simulink model "OFDM"  (R2022b)
settings: Solver=FixedStepDiscrete  StartTime=0.0  StopTime=inf  RelTol=1e-3
PreLoadFcn:
  | init
InitFcn:
  | init
values from neighbouring files (symbols this model uses):
  M = 3    [init.m]
  N = 2048    [init.m]
  nbPilots = 32    [init.m]
  nbZeros = N/8    (= 256)    [init.m]    (also in tests.m = N/8)
  nCycle = delayMax * N / Ts    (= 2)    [init.m]    (also in setMyParams.m = delaymax * n / Ts)
  nTotal = N + nCycle    (= 2050)    [init.m]    (also in setMyParams.m = n + nCycle)
  nUtile = N - ( nbZeros + nbPilots )    (= 1760)    [init.m]    (also in setMyParams.m = n - ( nbzeros + nbpilots ))
  Ts = N/B    (= 0.0001024)    [init.m]    (also in setMyParams.m = n/b)
undefined symbols (not defined in the file or in its folder): doppler, PSK
libraries: commchan3 x2, simulink x2, dspxfrm3 x2, commdigbbndam3 x2, commrandsrc3 x1, commsink2 x1
settings Model: SimulationMode=accelerator  Creator=pchabance  LastModifiedBy=AIIH
settings SolverCC: AlgebraicLoopSolver=TrustRegion  AutoInsertRateTranBlk=on
settings DataIOCC: LimitDataPoints=on  SaveOutput=off  SignalLogging=off  SaveTime=off  ReturnWorkspaceOutputs=off
settings OptimizationCC: EfficientMapNaN2IntZero=off  LifeSpan=inf
settings DebuggingCC: AlgebraicLoopMsg=error  SingleTaskRateTransMsg=error  UnconnectedInputMsg=warning  UnconnectedOutputMsg=warning  UnconnectedLineMsg=warning  AllowSymbolicDim=off  SFUnexpectedBacktrackingDiag=warning  SFNoUnconditionalDefaultTransitionDiag=warning  SFExecutionAtInitializationDiag=none  SFMachineParentedDataDiag=warning  ArithmeticOperatorsInVariantConditions=warning
settings HardwareCC: TargetBitPerPointer=64  TargetBitPerSizeT=64  TargetBitPerPtrDiffT=64  TargetLongLongMode=on  TargetIntDivRoundTo=Zero  TargetEndianess=LittleEndian  TargetWordSize=64  TargetHWDeviceType=MATLAB Host  ProdEqTarget=off
settings ModelReferenceCC: EnableRefExpFcnMdlSchedulingChecks=on
settings SFSimCC: SimUseLocalCustomCode=off  CustomCodeUndefinedFunction=UseInterfaceOnly
settings RTWCC: RTWUseLocalCustomCode=off
settings CodeAppCC: MaxIdLength=128  StateflowObjectComments=on
settings GRTTargetCC: TargetLangStandard=C89/C90 (ANSI)  CombineOutputUpdateFcns=off  GRTInterface=on

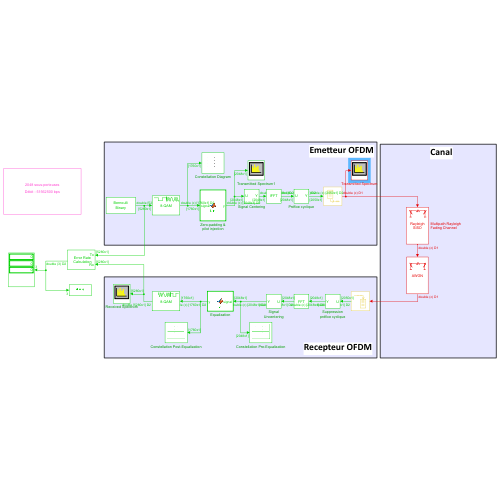
[thumbnail: Simulink's stored preview of the top-level diagram]
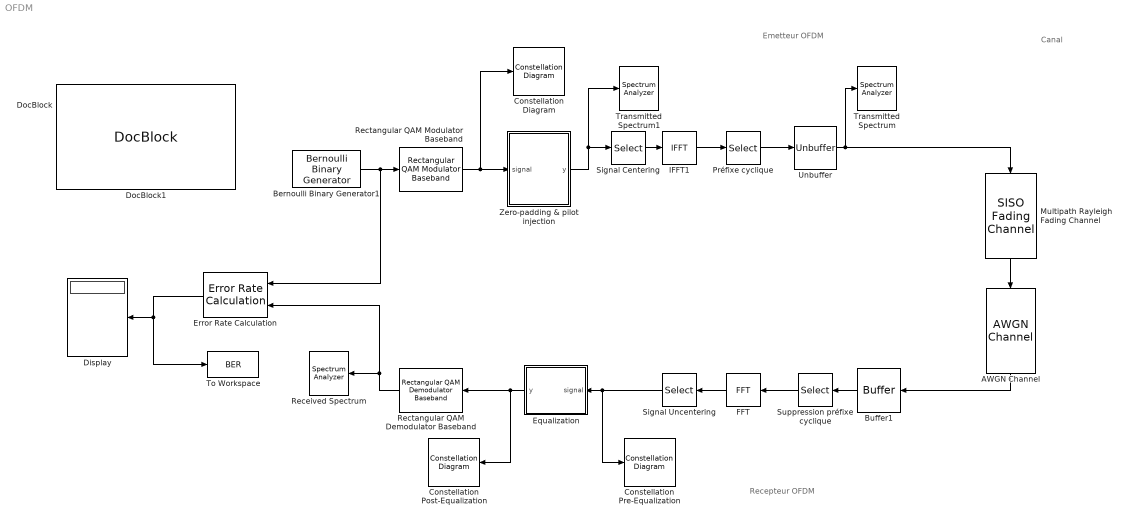
== system OFDM ==
  note: Emetteur OFDM
  note: Recepteur OFDM
  note: Canal
  AWGN Channel : commchan3/AWGN Channel  InputProcessing=Columns as channels (frame based)  seed=67  noiseMode="Signal to noise ratio  (SNR)"  EbNodB=10  EsNodB=30  SNRdB=SNR_  bitsPerSym=2  Ps=W  Tsym=256*5e-8  variance=1
  Bernoulli Binary Generator1 : commrandsrc3/Bernoulli Binary Generator  ProbabilityOfZero=0.5  SeedSource=Auto  Seed=0  SampleTime=Ts/(nUtile*M)  SamplesPerFrame=nUtile*M  OutputDataType=double  SimulateUsing=Code generation
  Buffer1 : Buffer  N=nTotal  OutputFrames=off
  Constellation Diagram : ConstellationDiagram  WindowPosition=[433.000000,362.000000,410.000000,300.000000,]  Visible=on  ScopeFrameLocation=window  DefaultConfigurationName=comm.scopes.ConstellationDiagramBlockCfg
  Constellation Post-Equalization : ConstellationDiagram  WindowPosition=[388.000000,174.000000,422.000000,306.000000,]  Visible=on  ScopeFrameLocation=window  SymbolsToDisplaySource=Property  SymbolsToDisplay=8000  ReferenceConstellation=8-PSK  XLimits=[-1.596 1.5905]  YLimits=[-1.9943 1.9888]  DefaultConfigurationName=comm.scopes.ConstellationDiagramBlockCfg
  Constellation Pre-Equalization : ConstellationDiagram  WindowPosition=[1.000000,26.000000,1280.000000,844.000000,]  Visible=on  ScopeFrameLocation=window  ReferenceConstellation=8-PSK  XLimits=[-2.0473 1.1549]  YLimits=[-2.4475 1.5551]  DefaultConfigurationName=comm.scopes.ConstellationDiagramBlockCfg
  Display : Display
  DocBlock : simulink/Model-Wide Utilities/DocBlock  DocumentType=Text
      content=|
      | Type your documentation here
  DocBlock1 : simulink/Model-Wide Utilities/DocBlock  DocumentType=Text  mask(DocBlock){}
      content=|
      | Type your documentation here
      mask Display:
      | % This is a new mask on top of the base mask.
      | % Use "View base mask" link below to see the base mask.
      | 
      | N = evalin('base','N');
      | fprintf([num2str(N),' sous-porteuses\n\n\n']);
      | 
      | rate = evalin('base','debit');
      | fprintf(['Débit : ',num2str(rate),' bps']);
  Equalization : MATLAB Function  TreatAsAtomicUnit=on
  Error Rate Calculation : commsink2/Error Rate Calculation  N=nUtile*M  st_delay=0  cp_mode=Entire frame  subframe=[]  PMode=Port  WsName=ErrorVec  RsMode2=off  stop=off  numErr=100  maxBits=1e6
  FFT : dspxfrm3/FFT  FFTImplementation=Auto  CompMethod=Table lookup  TableOpt=NEW  TableOptActive=Speed  BitRevOrder=off  Normalize=off  InheritFFTLength=on  FFTLength=64  WrapInput=on  roundingMode=Floor  overflowMode=off  firstCoeffDataTypeStr=Inherit: Same word length as input  firstCoeffLastDataTypeStr=Inherit: Same word length as input  outputMin=[]  outputMax=[]
  IFFT1 : dspxfrm3/IFFT  FFTImplementation=Auto  CompMethod=Table lookup  TableOpt=NEW  TableOptActive=Speed  BitRevOrder=off  cs_in=off  Normalize=on  InheritFFTLength=on  FFTLength=64  WrapInput=on  mode=Complex  outSamplingMode=Sample based  roundingMode=Floor  overflowMode=off  firstCoeffDataTypeStr=Inherit: Same word length as input  firstCoeffLastDataTypeStr=Inherit: Same word length as input  outputMin=[]  outputMax=[]
  Multipath Rayleigh Fading Channel : commchan3/SISO Fading Channel  InheritSampleRate=on  SampleRate=1  PathDelays=[0 0.5e-7 1e-7]  AveragePathGains=[0 -3 -6]  NormalizePathGains=on  FadingDistribution=Rayleigh  KFactor=3  DirectPathDopplerShift=0  DirectPathInitialPhase=0  MaximumDopplerShift=40  DopplerSpectrum=doppler('Jakes')  RandomStream=mt19937ar with seed  Seed=73  PathGainsOutputPort=off  ChannelFilterDelayOutputPort=off  SimulateUsing=Interpreted execution  Visualization=Off  PathsForDopplerDisplay=1  SamplesToDisplay=25%
  Préfixe cyclique : Selector  InputPortWidth=N  IndexOptions=Index vector (dialog)  Indices=[N-nCycle + 1:N 1:N]  OutputSizes=1
  Received Spectrum : SpectrumAnalyzer
  Rectangular QAM Demodulator Baseband : commdigbbndam3/Rectangular QAM Demodulator Baseband  M=2^M  OutType=Bit  DecType=Hard decision  VarSource=Dialog  Variance=1  Dec=Gray  Mapping=[0:15]  PowType=Average Power  MinDist=2  AvgPow=1  PeakPow=1  Ph=0  outDtype1=Inherit via internal rule  outDtype2=Inherit via internal rule  derotateFactorWordLen=16  derotateFactorDataTypeStr=Inherit: Same word length as input  derotateFactorLastDataTypeStr=Inherit: Same word length as input  denormFactorWordLen=16  denormFactorDataTypeStr=Inherit: Same word length as input  denormFactorLastDataTypeStr=Inherit: Same word length as input  prodOutWordLen=32  prodOutOverflowMode=Wrap  prodOutRoundingMode=Floor  prodOutOvFlMode=off  prodOutOvFlModeLastStrValue=off  sumWordLen=32
  Rectangular QAM Modulator Baseband : commdigbbndam3/Rectangular QAM Modulator Baseband  M=2^M  InType=Bit  Enc=Gray  Mapping=[0:15]  PowType=Average Power  MinDist=2  AvgPow=1  PeakPow=1  Ph=0  outDtype=double  outWordLen=16  outUDDataType=sfix(16)  outFracLenMode=Best precision  outFracLen=15  outDataTypeStr=double  outLastDataTypeStr=double
  Signal Uncentering : Selector  InputPortWidth=N  IndexOptions=Index vector (dialog)  Indices=[N/2+2:N 1:N/2+1]  OutputSizes=1
  Signal Centering : Selector  InputPortWidth=N  IndexOptions=Index vector (dialog)  Indices=[N/2:N 1:N/2-1]  OutputSizes=1
  Suppression préfixe cyclique : Selector  InputPortWidth=nTotal  IndexOptions=Index vector (dialog)  Indices=[nCycle+1:nTotal]  OutputSizes=1
  To Workspace : ToWorkspace  VariableName=BER  SaveFormat=Timeseries  SampleTime=-1
  Transmitted Spectrum : SpectrumAnalyzer
  Transmitted Spectrum1 : SpectrumAnalyzer
  Unbuffer : Unbuffer
  Zero-padding & pilot injection : MATLAB Function  TreatAsAtomicUnit=on
  wires:
  Rectangular QAM Modulator Baseband/1 -> Constellation Diagram/1, Zero-padding & pilot injection/1(signal)
  Signal Centering/1 -> IFFT1/1
  IFFT1/1 -> Préfixe cyclique/1
  Unbuffer/1 -> Multipath Rayleigh Fading Channel/1, Transmitted Spectrum/1
  FFT/1 -> Signal Uncentering/1
  Rectangular QAM Demodulator Baseband/1 -> Error Rate Calculation/2, Received Spectrum/1
  Error Rate Calculation/1 -> To Workspace/1, Display/1
  Bernoulli Binary Generator1/1 -> Rectangular QAM Modulator Baseband/1, Error Rate Calculation/1
  Signal Uncentering/1 -> Equalization/1(signal), Constellation Pre-Equalization/1
  Equalization/1(y) -> Rectangular QAM Demodulator Baseband/1, Constellation Post-Equalization/1
  Zero-padding & pilot injection/1(y) -> Transmitted Spectrum1/1, Signal Centering/1
  Multipath Rayleigh Fading Channel/1 -> AWGN Channel/1
  AWGN Channel/1 -> Buffer1/1
  Préfixe cyclique/1 -> Unbuffer/1
  Buffer1/1 -> Suppression préfixe cyclique/1
  Suppression préfixe cyclique/1 -> FFT/1

== matlab function OFDM/Equalization ==
  data: y output size=[nUtile,1]; signal input; nbPilots parameter; nUtile parameter; nbZeros parameter
function y = fcn(signal, nbPilots, nUtile, nbZeros)

    signalSansZeros = signal(nbZeros/2+1:nbZeros/2+nUtile+nbPilots);

    intervalle = floor(nUtile/nbPilots)+1;
    output = zeros(nUtile,1) + 1j * zeros(nUtile,1);
    indexOutput = 1;
    
    coeffs = zeros(nbPilots,1)+ 1j*zeros(nbPilots,1);
    indexCoeffs = 1;
    indexes = zeros(nbPilots,1);
    indexIndexes = 1;
    
    for i = 1:nUtile+nbPilots
        if mod(i+floor(intervalle/2),intervalle) == 0
            if (indexCoeffs <= nbPilots)
                coeffs(indexCoeffs) = (sqrt(2)+sqrt(2)*1j)/signalSansZeros(i);
                indexes(indexIndexes) = i;
                indexCoeffs = indexCoeffs + 1;
                indexIndexes = indexIndexes + 1;
            end
        end
    end
    
    coeffsInterp = interp1(indexes,coeffs,1:nUtile+nbPilots,'spline');
    
    coeffsInterp(1:intervalle) = coeffs(1);
    coeffsInterp(nUtile+nbPilots-intervalle:end) = coeffs(nbPilots);
    
    for i = 1:nUtile+nbPilots
        if mod(i+floor(intervalle/2),intervalle) ~= 0
            output(indexOutput) = signalSansZeros(i)*coeffsInterp(i);
            indexOutput = indexOutput + 1;
        end
    end

y = output;

== matlab function OFDM/Zero-padding & pilot injection ==
  data: y output size=[N,1]; nbZeros parameter; nbPilots parameter; signal input size=nUtile; nUtile parameter
function y = fcn(nbZeros, nbPilots, signal, nUtile)

    index = 1;
    
    intervalle = floor(nUtile/nbPilots)+1;
    output = zeros(nbZeros+nbPilots+nUtile,1)+1j * zeros(nbZeros+nbPilots+nUtile,1);
    
    for i=nbZeros/2+1:nUtile+nbZeros/2+nbPilots
        if mod(i-nbZeros/2+floor(intervalle/2),intervalle) == 0
            output(i)= sqrt(2)+sqrt(2)*1j;
        else
            output(i)=signal(index);
            index = index+1;
        end
    end
y = output;
